simulink subsystem "PT1"  (R2023b)
settings: Solver=VariableStepAuto  StartTime=0.0  StopTime=10.0  RelTol=1e-3
settings Model: Creator=Alex  LastModifiedBy=Alex

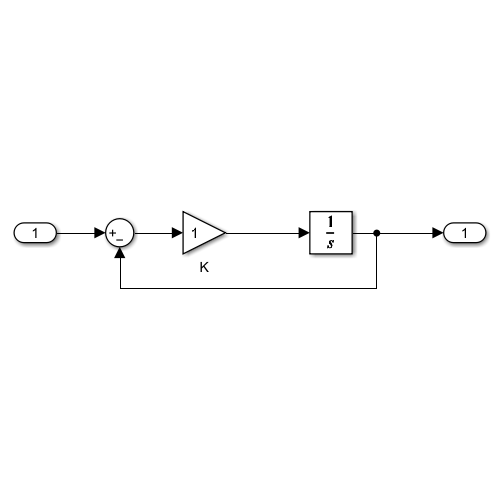
[thumbnail: Simulink's stored preview of the top-level diagram]
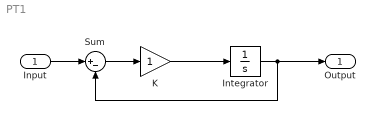
== system PT1 ==
  Input : Inport
  Integrator : Integrator
  K : Gain
  Sum : Sum  Inputs=|+-
  Output : Outport
  wires:
  Input/1 -> Sum/1
  Integrator/1 -> Sum/2, Output/1
  Sum/1 -> K/1
  K/1 -> Integrator/1
